simulink model "DC_Motor_Control_PM_2019a"  (R2021a)
settings: Solver=ode23s  StartTime=0.0  StopTime=0.2  RelTol=1e-3  EnableMultiTasking=on
undefined symbols (not defined in the file): B, J, K_m, K_t, ki_curr, ki_speed, kp_curr, kp_speed, La, Ra
libraries: slpidlib x1
settings Model: Creator=matti  LastModifiedBy=arco
settings SolverCC: AlgebraicLoopSolver=TrustRegion
settings DataIOCC: LimitDataPoints=on  SaveFormat=Array  ReturnWorkspaceOutputs=off
settings OptimizationCC: LifeSpan=inf
settings DebuggingCC: SolverPrmCheckMsg=warning  SFUnexpectedBacktrackingDiag=warning  SFNoUnconditionalDefaultTransitionDiag=warning  SFExecutionAtInitializationDiag=none  SFMachineParentedDataDiag=warning  ArithmeticOperatorsInVariantConditions=warning
settings HardwareCC: ProdBitPerPointer=32  ProdBitPerSizeT=32  ProdBitPerPtrDiffT=32  ProdLargestAtomicFloat=None  ProdIntDivRoundTo=Undefined  ProdEndianess=Unspecified  ProdWordSize=32  ProdHWDeviceType=32-bit Generic
settings ModelReferenceCC: PropagateSignalLabelsOutOfModel=off
settings SFSimCC: SimUseLocalCustomCode=off  CustomCodeUndefinedFunction=UseInterfaceOnly
settings RTWCC: RTWUseLocalCustomCode=off
settings CodeAppCC: StateflowObjectComments=on
settings GRTTargetCC: TargetLangStandard=C89/C90 (ANSI)
settings ConfigComp: CovMetricSettings=dw  CovSaveCumulativeToWorkspaceVar=on  CovSaveSingleToWorkspaceVar=on  CovExternalEMLEnable=off  CovSFcnEnable=off

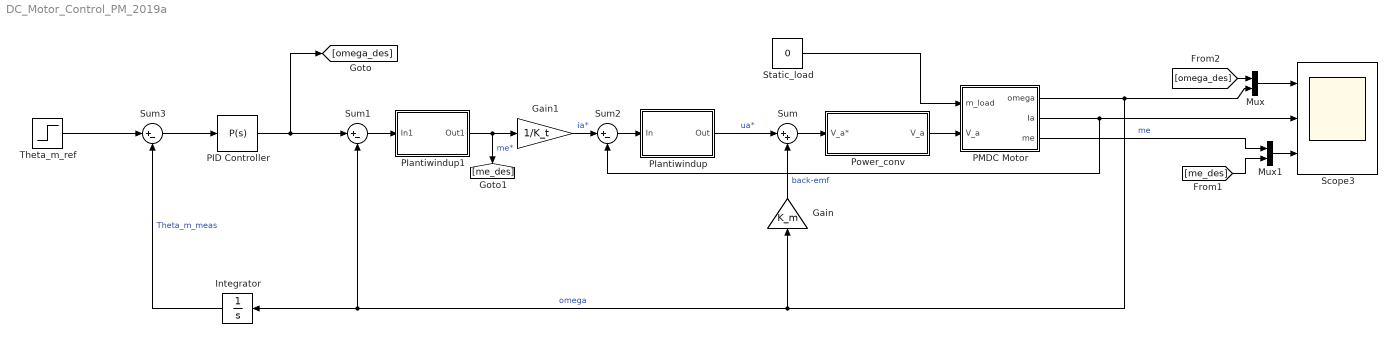
== system DC_Motor_Control_PM_2019a ==
  Gain : Gain  Gain=K_m
  Gain1 : Gain  Gain=1/K_t
  Integrator : Integrator
  Mux : Mux  Inputs=2
  Mux1 : Mux  Inputs=2
  PID Controller : slpidlib/PID Controller  Controller=P  Form=Parallel  TimeDomain=Continuous-time  UseExternalTs=off  SampleTime=-1  IntegratorMethod=Forward Euler  FilterMethod=Forward Euler  ControllerParametersSource=internal  P=1  I=1  D=0  UseFilter=on  N=100  TunerSelectOption=Transfer Function Based (PID Tuner App)  InitialConditionSource=internal  InitialConditionForIntegrator=0  InitialConditionForFilter=0  DifferentiatorICPrevScaledInput=0  ExternalReset=none  TrackingMode=off  Kt=1  LimitOutput=off  SatLimitsSource=internal  UpperSaturationLimit=inf  LowerSaturationLimit=-inf  LinearizeAsGain=on  AntiWindupMode=none  Kb=1  POutMin=[]  POutMax=[]  IOutMin=[]  IOutMax=[]  DOutMin=[]  DOutMax=[]  NOutMin=[]  NOutMax=[]  SumOutMin=[]  SumOutMax=[]  SaturationOutMin=[]  SaturationOutMax=[]  PParamMin=[]  PParamMax=[]  IParamMin=[]  IParamMax=[]  DParamMin=[]  DParamMax=[]  NParamMin=[]  NParamMax=[]  KbParamMin=[]  KbParamMax=[]  KtParamMin=[]  KtParamMax=[]  KbOutMin=[]  KbOutMax=[]  KtOutMin=[]  KtOutMax=[]  IntegratorOutMin=[]  IntegratorOutMax=[]  FilterOutMin=[]  FilterOutMax=[]  SumI1OutMin=[]  SumI1OutMax=[]  SumI2OutMin=[]  SumI2OutMax=[]  SumI3OutMin=[]  SumI3OutMax=[]  SumI4OutMin=[]  SumI4OutMax=[]  SumDOutMin=[]  SumDOutMax=[]  DifferentiatorOutMin=[]  DifferentiatorOutMax=[]  FilterDiffOutCoefMin=[]  FilterDiffOutCoefMax=[]  ReciprocalOutMin=[]  ReciprocalOutMax=[]  SumDenOutMin=[]  SumDenOutMax=[]  SumNumOutMin=[]  SumNumOutMax=[]  DivideOutMin=[]  DivideOutMax=[]  UdiffTsProdOutMin=[]  UdiffTsProdOutMax=[]  NTsProdOutMin=[]  NTsProdOutMax=[]  UintegralTsProdOutMin=[]  UintegralTsProdOutMax=[]  UngainTsProdOutMin=[]  UngainTsProdOutMax=[]  IntegratorContinuousStateAttributes=''  IntegratorStateMustResolveToSignalObject=off  IntegratorRTWStateStorageClass=Auto  FilterContinuousStateAttributes=''  FilterStateMustResolveToSignalObject=off  FilterRTWStateStorageClass=Auto  ParallelPVariant=InternalParameters  IdealPVariant=Disabled  IVariant=Disabled  DVariant=Disabled  IntegratorVariant=Disabled  SatVariant=Disabled  AWVariant=Disabled  PCopyVariant=Disabled  TRVariant=Disabled  FdbkBlocksVariant=Forward  IdealPFdbkVariant=Disabled  SatFdbkVariant=Disabled  DerivativeFilterVariant=Disabled  NVariant=Disabled  NCopyVariant=Disabled_SignalSpec  FilterICVariant=Disabled  IntegratorICVariant=Disabled  ExternalResetVariant=Disabled  TRSumVariant=Passthrough  SumFdbkVariant=Disabled  SumVariant=Passthrough_P  TsampFilterVariant=InternalTs  TsampNgainVariant=Passthrough  TsampIntegralVariant=Disabled_SignalSpec  ExternalSaturationOutDataTypeStr=Inherit: Same as second input
  PIantiwindup : Subsystem  mask{Kp=kp_curr, Ki=ki_curr, sat_up=600, sat_down=-600}
      mask prompts: sat_up "Upper sat. limit"; sat_down "Lower Sat. Limit"
      mask Display: disp('current\ncontroller\n(PI)')
  PIantiwindup1 : Subsystem  mask{Kp=kp_speed, Ki=ki_speed, sat_up=1000, sat_down=-1000}
      mask prompts: sat_up "Upper sat. limit"; sat_down "Lower Sat. Limit"
      mask Display: disp('speed\ncontroller\n(PI)')
  PMDC Motor : Subsystem
  Power_conv : Subsystem
  Scope3 : Scope  NumInputPorts=3
  Static_load : Constant  Value=0
  Sum : Sum  Inputs=|++
  Sum1 : Sum  Inputs=|+-
  Sum2 : Sum  Inputs=|+-
  Sum3 : Sum  Inputs=|+-
  Theta_m_ref : Step  SampleTime=0
  wires:
  PMDC Motor/1(omega) -> Gain/1, Sum1/2, Integrator/1, Mux/2  "omega"
  PIantiwindup/1(Out) -> Sum/1  "ua*"
  Sum2/1 -> PIantiwindup/1(In)
  PIantiwindup1/1(Out1) -> [me_des], Gain1/1  "me*"
  PID Controller/1 -> Sum1/1, [omega_des]
  Sum1/1 -> PIantiwindup1/1(In1)
  PMDC Motor/2(Ia) -> Sum2/2, Scope3/2
  PMDC Motor/3(me) -> Mux1/1  "me"
  Gain/1 -> Sum/2  "back-emf"
  Gain1/1 -> Sum2/1  "ia*"
  Mux/1 -> Scope3/1
  [me_des] -> Mux1/2
  Mux1/1 -> Scope3/3
  [omega_des] -> Mux/1
  Static_load/1 -> PMDC Motor/1(m_load)
  Sum/1 -> Power_conv/1(V_a*)
  Power_conv/1(V_a) -> PMDC Motor/2(V_a)
  Integrator/1 -> Sum3/2  "Theta_m_meas"
  Sum3/1 -> PID Controller/1
  Theta_m_ref/1 -> Sum3/1

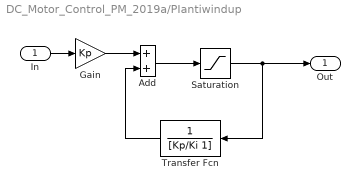
== system DC_Motor_Control_PM_2019a/PIantiwindup ==
  In : Inport
  Add : Sum
  Gain : Gain  Gain=Kp
  Saturation : Saturate  UpperLimit=sat_up  LowerLimit=sat_down
  Transfer Fcn : TransferFcn  Denominator=[Kp/Ki 1]
  Out : Outport  VectorParamsAs1DForOutWhenUnconnected=off
  wires:
  Saturation/1 -> Out/1, Transfer Fcn/1
  In/1 -> Gain/1
  Gain/1 -> Add/1
  Add/1 -> Saturation/1
  Transfer Fcn/1 -> Add/2

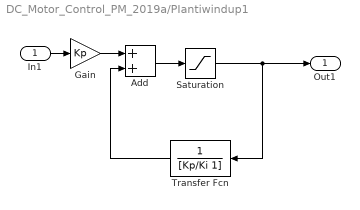
== system DC_Motor_Control_PM_2019a/PIantiwindup1 ==
  In1 : Inport
  Add : Sum
  Gain : Gain  Gain=Kp
  Saturation : Saturate  UpperLimit=sat_up  LowerLimit=sat_down
  Transfer Fcn : TransferFcn  Denominator=[Kp/Ki 1]
  Out1 : Outport  VectorParamsAs1DForOutWhenUnconnected=off
  wires:
  Transfer Fcn/1 -> Add/2
  Add/1 -> Saturation/1
  Gain/1 -> Add/1
  In1/1 -> Gain/1
  Saturation/1 -> Transfer Fcn/1, Out1/1

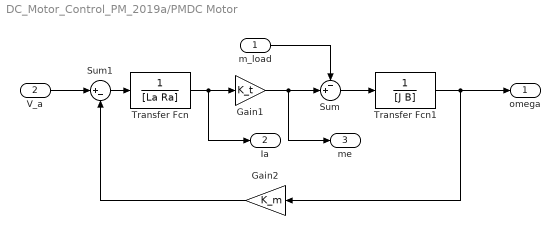
== system DC_Motor_Control_PM_2019a/PMDC Motor ==
  m_load : Inport
  V_a : Inport  Port=2
  Gain1 : Gain  Gain=K_t
  Gain2 : Gain  Gain=K_m
  Sum : Sum  Inputs=-+|
  Sum1 : Sum  Inputs=|+-
  Transfer Fcn : TransferFcn  Denominator=[La Ra]
  Transfer Fcn1 : TransferFcn  Denominator=[J B]
  omega : Outport  VectorParamsAs1DForOutWhenUnconnected=off
  Ia : Outport  Port=2  VectorParamsAs1DForOutWhenUnconnected=off
  me : Outport  Port=3  VectorParamsAs1DForOutWhenUnconnected=off
  wires:
  m_load/1 -> Sum/1
  Gain2/1 -> Sum1/2
  Sum1/1 -> Transfer Fcn/1
  Gain1/1 -> me/1, Sum/2
  Transfer Fcn/1 -> Ia/1, Gain1/1
  Transfer Fcn1/1 -> omega/1, Gain2/1
  Sum/1 -> Transfer Fcn1/1
  V_a/1 -> Sum1/1

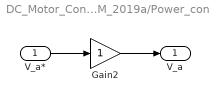
== system DC_Motor_Control_PM_2019a/Power_conv ==
  V_a* : Inport
  Gain2 : Gain
  V_a : Outport
  wires:
  V_a*/1 -> Gain2/1
  Gain2/1 -> V_a/1
